simulink model "a3_4_example_exponential"  (R2018a)
settings: Solver=VariableStepAuto  StartTime=0.0  StopTime=10.0  RelTol=1e-3
settings Model: Creator=r0x6f736f646f  LastModifiedBy=r0x6f736f646f

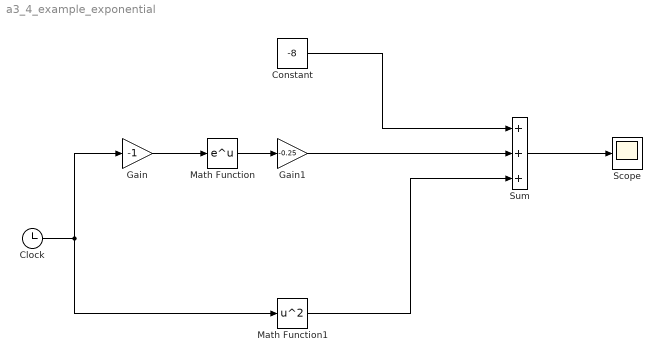
== system a3_4_example_exponential ==
  Clock : Clock
  Constant : Constant  Value=-8
  Gain : Gain  Gain=-1
  Gain1 : Gain  Gain=-0.25
  Math Function : Math  SaturateOnIntegerOverflow=on
  Math Function1 : Math  Operator=square  SaturateOnIntegerOverflow=on
  Scope : Scope
  Sum : Sum  Inputs=+++
  wires:
  Gain/1 -> Math Function/1
  Clock/1 -> Gain/1, Math Function1/1
  Constant/1 -> Sum/1
  Math Function1/1 -> Sum/3
  Math Function/1 -> Gain1/1
  Gain1/1 -> Sum/2
  Sum/1 -> Scope/1
